simulink model "energy_aware_controller_v2"  (R2020b)
settings: Solver=VariableStepAuto  StartTime=0.0  StopTime=42  RelTol=1e-3
values from neighbouring files (symbols this model uses):
  b0 = 2 * sqrt(k0 * m_R)    [compliance_PLUS_energy_setup.m]    (also in compliance_adjusting_setup.m = 2; energy_aware_setup.m = 20; optim_criteria.m = 0.2; plot_meshes.m = 0.2)
  E_max = 1    [compliance_PLUS_energy_setup.m]    (also in energy_aware_setup.m = 0.7; optim_criteria.m = 0.5; plot_meshes.m = 0.5; setup.m)
  k0 = 20    [compliance_PLUS_energy_setup.m]    (also in compliance_adjusting_setup.m = 10; energy_aware_setup.m = 100; optim_criteria.m = 1; plot_meshes.m = 1)
  km = 100    [compliance_PLUS_energy_setup.m]    (also in compliance_adjusting_setup.m; energy_aware_setup.m; setup.m)
  m_R = 1    [compliance_PLUS_energy_setup.m]    (also in compliance_adjusting_setup.m; energy_aware_setup.m; setup.m)
  P_max = 1    [compliance_PLUS_energy_setup.m]    (also in energy_aware_setup.m = 0.2; optim_criteria.m = 0.5; plot_meshes.m = 0.5; setup.m = 0.1)
  s0 = 5    [compliance_PLUS_energy_setup.m]    (also in energy_aware_setup.m; setup.m)
  t_collision = 20    [compliance_PLUS_energy_setup.m]    (also in compliance_adjusting_setup.m; energy_aware_setup.m; setup.m)
  t_init = 2    [compliance_PLUS_energy_setup.m]    (also in compliance_adjusting_setup.m; energy_aware_setup.m; setup.m)
  x_O = 0.5    [compliance_PLUS_energy_setup.m]    (also in compliance_adjusting_setup.m; energy_aware_setup.m; setup.m)
  x_O2 = -2    [compliance_PLUS_energy_setup.m]    (also in compliance_adjusting_setup.m)
  x_R = 0    [compliance_PLUS_energy_setup.m]    (also in compliance_adjusting_setup.m; energy_aware_setup.m; setup.m)
settings Model: Creator=kika  LastModifiedBy=kika

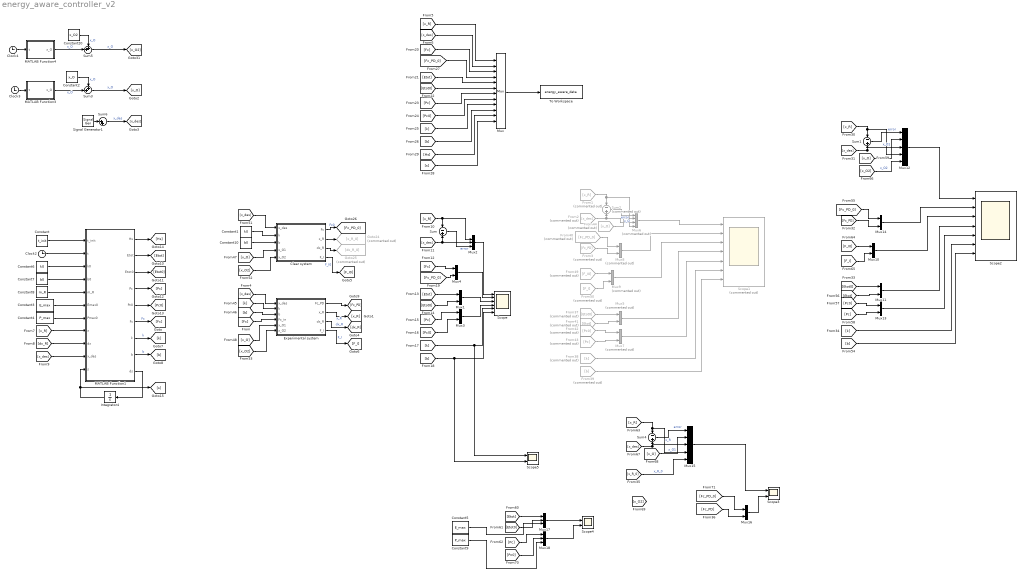
== system energy_aware_controller_v2 ==
  Clear system : Subsystem
  Clock2 : Clock
  Clock3 : Clock
  Clock4 : Clock
  Constant : Constant  Value=t_init
  Constant1 : Constant  Value=k0
  Constant10 : Constant  Value=b0
  Constant2 : Constant  Value=x_O
  Constant20 : Constant  Value=x_O2
  Constant3 : Constant  Value=E_max
  Constant4 : Constant  Value=P_max
  Constant5 : Constant  Value=E_max
  Constant6 : Constant  Value=k0
  Constant7 : Constant  Value=b0
  Constant8 : Constant  Value=m_R
  Constant9 : Constant  Value=P_max
  Experimental system : Subsystem
  From1 : From  Commented=on  GotoTag=x_R
  From2 : From  Commented=on  GotoTag=x_des
  From3 : From  Commented=on  GotoTag=Fc_PD
  From37 : From  Commented=on  GotoTag=Etot0
  From38 : From  Commented=on  GotoTag=k
  From39 : From  Commented=on  GotoTag=b
  From40 : From  Commented=on  GotoTag=Fc_PD_0
  From41 : From  Commented=on  GotoTag=Etot
  From42 : From  Commented=on  GotoTag=Pc0
  From43 : From  Commented=on  GotoTag=Pc
  From44 : From  Commented=on  GotoTag=x_O
  From49 : From  Commented=on  GotoTag=F_I0
  From50 : From  Commented=on  GotoTag=F_I
  Goto24 : Goto  Commented=on  GotoTag=x_R_0
  Goto25 : Goto  Commented=on  GotoTag=dx_R_0
  Integrator4 : Integrator  InitialCondition=s0
  MATLAB Function1 : MATLAB Function  TreatAsAtomicUnit=on
  MATLAB Function3 : MATLAB Function  TreatAsAtomicUnit=on
  MATLAB Function4 : MATLAB Function  TreatAsAtomicUnit=on
  Mux : Mux  Inputs=12
  Mux{1,3..4,10..11,13..14,16} (8 alike) : Mux  Inputs=2
  Mux12 : Mux  Inputs=5
  Mux15 : Mux  Inputs=5
  Mux17 : Mux  Inputs=3
  Mux18 : Mux  Inputs=3
  Mux2 : Mux  Inputs=3
  Mux{5,7..9} (4 alike) : Mux  Commented=on  Inputs=2
  Mux6 : Mux  Commented=on
  Scope : Scope  NumInputPorts=6
  Scope1 : Scope  Commented=on  NumInputPorts=7
  Scope2 : Scope  NumInputPorts=7
  Scope3 : Scope  NumInputPorts=2
  Scope4 : Scope  NumInputPorts=2
  Scope5 : Scope  NumInputPorts=2
  Signal Generator1 : SignalGenerator  Frequency=0.5  Units=rad/sec
  Sum : Sum  Inputs=-+
  Sum1 : Sum  Inputs=-+
  Sum2 : Sum  Commented=on  Inputs=-+
  Sum3 : Sum  Inputs=++|
  Sum4 : Sum  Inputs=-+
  Sum5 : Sum  Inputs=++|
  Sum6 : Sum  Inputs=|++
  To Workspace : ToWorkspace  VariableName=energy_aware_data  SaveFormat=Timeseries  SampleTime=-1
  wires:
  Constant4/1 -> MATLAB Function1/7(Pmax0)
  Constant3/1 -> MATLAB Function1/6(Emax0)
  MATLAB Function1/9(ds) -> Integrator4/1
  Constant7/1 -> MATLAB Function1/4(b0)
  MATLAB Function1/7(k) -> [k]  "k"
  Constant8/1 -> MATLAB Function1/5(m_R)
  Constant6/1 -> MATLAB Function1/3(k0)
  Integrator4/1 -> MATLAB Function1/11(s), [s]
  Clock2/1 -> MATLAB Function1/2(t)
  MATLAB Function1/8(b) -> [b]  "b"
  Constant/1 -> MATLAB Function1/1(t_init)
  MATLAB Function1/6(Fc) -> [Fc]  "Fc"
  [dx_R] -> MATLAB Function1/9(dx)
  [x_R] -> MATLAB Function1/8(x)
  [x_des] -> MATLAB Function1/10(x_des)
  [x_R] -> Sum/1, Mux2/1
  [x_des] -> Mux2/2, Sum/2
  Mux2/1 -> Scope/1
  [Fc] -> Mux4/1
  MATLAB Function1/5(Pc0) -> [Pc0]
  MATLAB Function1/4(Pc) -> [Pc]
  MATLAB Function1/3(Etot0) -> [Etot0]
  MATLAB Function1/2(Etot) -> [Etot]
  MATLAB Function1/1(Hs) -> [Hs]
  [Etot] -> Mux1/1
  [Etot0] -> Mux1/2
  [Pc0] -> Mux3/2
  [Pc] -> Mux3/1
  Mux1/1 -> Scope/3
  Mux3/1 -> Scope/4
  [k] -> Scope5/1, Scope/5
  [b] -> Scope5/2, Scope/6
  [Fc_PD_0] -> Mux4/2
  Mux4/1 -> Scope/2
  Sum/1 -> Mux2/3  "error"
  [Fc_PD_0] -> Mux/4
  [Fc] -> Mux/3
  [Etot] -> Mux/5
  [Etot0] -> Mux/6
  [x_des] -> Mux/2
  [x_R] -> Mux/1
  [Pc] -> Mux/7
  [Pc0] -> Mux/8
  [k] -> Mux/9
  [b] -> Mux/10
  Mux/1 -> To Workspace/1
  [Hs] -> Mux/11
  [s] -> Mux/12
  From37/1 -> Mux5/1
  Mux7/1 -> Scope1/5
  Mux8/1 -> Scope1/2
  Mux6/1 -> Scope1/1
  From43/1 -> Mux7/2
  Mux9/1 -> Scope1/3
  From42/1 -> Mux7/1
  From1/1 -> Mux6/4, Sum2/1
  From50/1 -> Mux9/2
  From41/1 -> Mux5/2
  From40/1 -> Mux8/1
  From49/1 -> Mux9/1
  From38/1 -> Scope1/6
  From39/1 -> Scope1/7
  Sum2/1 -> Mux6/1  "error"
  From3/1 -> Mux8/2
  Mux5/1 -> Scope1/4
  From44/1 -> Mux6/2  "x_O"
  From2/1 -> Mux6/3, Sum2/2
  Sum6/1 -> [x_des]  "x_des"
  Clock4/1 -> MATLAB Function4/1(t)
  Clock3/1 -> MATLAB Function3/1(t)
  Constant20/1 -> Sum5/1  "x_O"
  MATLAB Function4/1(x_O) -> Sum5/2  "x_O"
  MATLAB Function3/1(x_O) -> Sum3/2  "x_O"
  Sum5/1 -> [x_O2]  "x_O"
  Constant2/1 -> Sum3/1  "x_O"
  Sum3/1 -> [x_O]  "x_O"
  Signal Generator1/1 -> Sum6/1
  Constant10/1 -> Clear system/3(b)
  Constant1/1 -> Clear system/2(k)
  [b] -> Experimental system/3(b)
  [x_des] -> Clear system/1(x_des)
  Clear system/3(dx_R) -> Goto25/1
  [x_des] -> Experimental system/1(x_des)
  [k] -> Experimental system/2(k)
  Clear system/1(Fc) -> [Fc_PD_0]  "Fc0"
  Experimental system/3(dx_R) -> [dx_R]  "dx_R"
  Clear system/4(F_I) -> [F_I0]  "F_I0"
  [x_O2] -> Experimental system/6(x_O2)
  [Fc] -> Experimental system/4(Fc_in)
  [x_O] -> Experimental system/5(x_O1)
  [x_O] -> Clear system/4(x_O1)
  [x_O2] -> Clear system/5(x_O2)
  Clear system/2(x_R) -> Goto24/1
  Experimental system/1(Fc_PD) -> [Fc_PD]
  Experimental system/2(x_R) -> [x_R]  "x_R"
  Experimental system/4(F_I) -> [F_I]  "F_I"
  Mux14/1 -> Scope2/2
  [x_R] -> Mux12/4, Sum1/1
  Mux12/1 -> Scope2/1
  [b] -> Scope2/7
  [Pc] -> Mux13/2
  [F_I] -> Mux10/2
  Sum1/1 -> Mux12/1  "error"
  [F_I0] -> Mux10/1
  [x_des] -> Mux12/3, Sum1/2
  [x_O2] -> Mux12/5  "x_O2"
  [x_O] -> Mux12/2  "x_O1"
  [k] -> Scope2/6
  [Etot] -> Mux11/2
  Mux13/1 -> Scope2/5
  [Fc_PD] -> Mux14/2
  [Pc0] -> Mux13/1
  Mux11/1 -> Scope2/4
  [Fc_PD_0] -> Mux14/1
  Mux10/1 -> Scope2/3
  [Etot0] -> Mux11/1
  [x_R] -> Mux15/4, Sum4/1  "x_R"
  [x_O] -> Mux15/2  "x_O1"
  Sum4/1 -> Mux15/1  "error"
  Mux15/1 -> Scope3/1
  [x_des] -> Mux15/3, Sum4/2
  [Fc_PD_0] -> Mux16/1
  [x_R_0] -> Mux15/5  "x_R_0"
  [Fc_PD] -> Mux16/2
  Mux16/1 -> Scope3/2
  Mux18/1 -> Scope4/2
  [Pc0] -> Mux18/2
  [Etot] -> Mux17/1
  [Etot0] -> Mux17/2
  Mux17/1 -> Scope4/1
  [Pc] -> Mux18/1
  Constant5/1 -> Mux17/3
  Constant9/1 -> Mux18/3

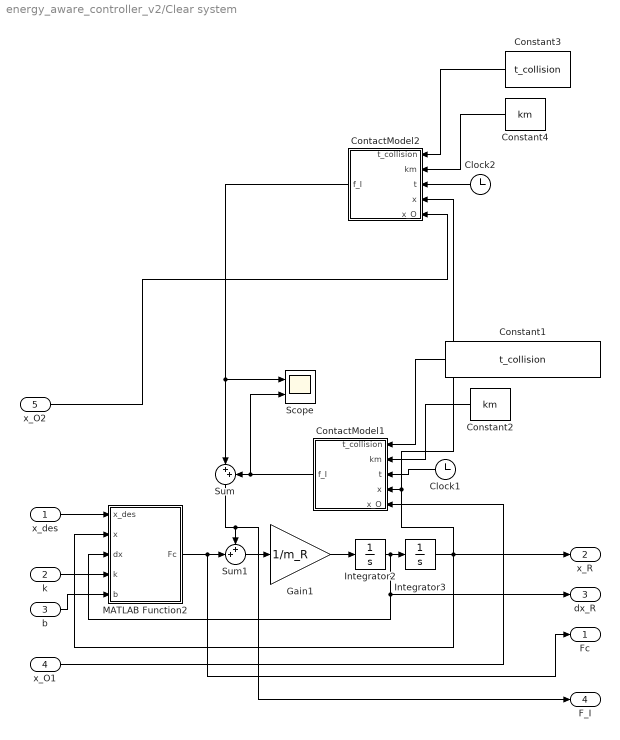
== system energy_aware_controller_v2/Clear system ==
  x_des : Inport
  k : Inport  Port=2
  b : Inport  Port=3
  x_O1 : Inport  Port=4
  x_O2 : Inport  Port=5
  Clock1 : Clock
  Clock2 : Clock
  Constant1 : Constant  Value=t_collision
  Constant2 : Constant  Value=km
  Constant3 : Constant  Value=t_collision
  Constant4 : Constant  Value=km
  ContactModel1 : MATLAB Function  TreatAsAtomicUnit=on
  ContactModel2 : MATLAB Function  TreatAsAtomicUnit=on
  Gain1 : Gain  Gain=1/m_R
  Integrator2 : Integrator
  Integrator3 : Integrator  InitialCondition=x_R
  MATLAB Function2 : MATLAB Function  TreatAsAtomicUnit=on
  Scope : Scope  NumInputPorts=2
  Sum : Sum  Inputs=|++
  Sum1 : Sum  Inputs=++|
  Fc : Outport
  x_R : Outport  Port=2
  dx_R : Outport  Port=3
  F_I : Outport  Port=4
  wires:
  k/1 -> MATLAB Function2/4(k)
  ContactModel1/1(f_I) -> Scope/2, Sum/2
  Clock1/1 -> ContactModel1/3(t)
  x_des/1 -> MATLAB Function2/1(x_des)
  b/1 -> MATLAB Function2/5(b)
  Sum1/1 -> Gain1/1
  x_O1/1 -> ContactModel1/5(x_O)
  Gain1/1 -> Integrator2/1
  MATLAB Function2/1(Fc) -> Fc/1, Sum1/2
  Integrator2/1 -> dx_R/1, MATLAB Function2/3(dx), Integrator3/1
  Constant1/1 -> ContactModel1/1(t_collision)
  Constant2/1 -> ContactModel1/2(km)
  Constant3/1 -> ContactModel2/1(t_collision)
  Integrator3/1 -> x_R/1, ContactModel2/4(x), ContactModel1/4(x), MATLAB Function2/2(x)
  x_O2/1 -> ContactModel2/5(x_O)
  Constant4/1 -> ContactModel2/2(km)
  Clock2/1 -> ContactModel2/3(t)
  Sum/1 -> F_I/1, Sum1/1
  ContactModel2/1(f_I) -> Sum/1, Scope/1

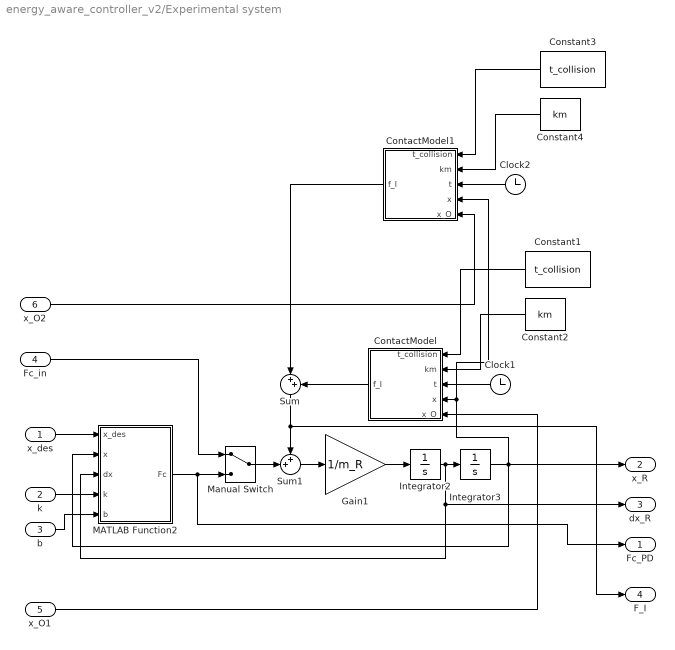
== system energy_aware_controller_v2/Experimental system ==
  x_des : Inport
  k : Inport  Port=2
  b : Inport  Port=3
  Fc_in : Inport  Port=4
  x_O1 : Inport  Port=5
  x_O2 : Inport  Port=6
  Clock1 : Clock
  Clock2 : Clock
  Constant1 : Constant  Value=t_collision
  Constant2 : Constant  Value=km
  Constant3 : Constant  Value=t_collision
  Constant4 : Constant  Value=km
  ContactModel : MATLAB Function  TreatAsAtomicUnit=on
  ContactModel1 : MATLAB Function  TreatAsAtomicUnit=on
  Gain1 : Gain  Gain=1/m_R
  Integrator2 : Integrator
  Integrator3 : Integrator  InitialCondition=x_R
  MATLAB Function2 : MATLAB Function  TreatAsAtomicUnit=on
  Manual Switch : ManualSwitch
  Sum : Sum  Inputs=|++
  Sum1 : Sum  Inputs=++|
  Fc_PD : Outport
  x_R : Outport  Port=2
  dx_R : Outport  Port=3
  F_I : Outport  Port=4
  wires:
  k/1 -> MATLAB Function2/4(k)
  ContactModel/1(f_I) -> Sum/2
  Clock1/1 -> ContactModel/3(t)
  Integrator3/1 -> x_R/1, ContactModel1/4(x), ContactModel/4(x), MATLAB Function2/2(x)
  x_des/1 -> MATLAB Function2/1(x_des)
  b/1 -> MATLAB Function2/5(b)
  Sum1/1 -> Gain1/1
  x_O1/1 -> ContactModel/5(x_O)
  Gain1/1 -> Integrator2/1
  MATLAB Function2/1(Fc) -> Manual Switch/2, Fc_PD/1
  Integrator2/1 -> dx_R/1, MATLAB Function2/3(dx), Integrator3/1
  Constant1/1 -> ContactModel/1(t_collision)
  Constant2/1 -> ContactModel/2(km)
  Fc_in/1 -> Manual Switch/1
  Manual Switch/1 -> Sum1/2
  ContactModel1/1(f_I) -> Sum/1
  Constant4/1 -> ContactModel1/2(km)
  Constant3/1 -> ContactModel1/1(t_collision)
  Clock2/1 -> ContactModel1/3(t)
  x_O2/1 -> ContactModel1/5(x_O)
  Sum/1 -> F_I/1, Sum1/1

== matlab function energy_aware_controller_v2/MATLAB Function4 ==
  data: t input; x_O output
function x_O = fcn(t)

    x_O = 0;
    if t > 56 && t < 65
        x_O = sin(0.5 * t + pi) + 0.5;
    end
    if t > 71 && t < 85
        x_O = 1.5;
    end
%     if t >= 44.5 && t < 46.8
%         x_O = 3*sin(1.5 * t - pi/4);
%     end

== matlab function energy_aware_controller_v2/Experimental system/ContactModel1 ==
  data: t_collision input; km input; t input; f_I output; x input; x_O input
function f_I = fcn(t_collision, km, t, x, x_O)


f_I = 0;

if t > t_collision
    if x < x_O
        f_I = km * (x_O - x);
    end
end

== matlab function energy_aware_controller_v2/Experimental system/MATLAB Function2 ==
  data: x_des input; Fc output; x input; dx input; k input; b input
function Fc = fcn(x_des, x, dx, k, b)

Fc = k * (x_des - x) - b * dx;

== matlab function energy_aware_controller_v2/Experimental system/ContactModel ==
  data: t_collision input; km input; t input; f_I output; x input; x_O input
function f_I = fcn(t_collision, km, t, x, x_O)


f_I = 0;

if t > t_collision
    if x > x_O
        f_I = km * (x_O - x);
    end
end

% if t > t_collision
%     if abs(x) - abs(x_O) > 0
%         f_I = km * (abs(x_O) - abs(x));
%     end
% end

== matlab function energy_aware_controller_v2/MATLAB Function3 ==
  data: t input; x_O output
function x_O = fcn(t)

    offset = -0.3;
    x_O = 1;
    if t > 23 && t < 35
        x_O = sin(0.5 * t + pi);
    end
    if t >= offset + 44.5 && t < offset +46.8
        x_O = 2*sin(1.5 * t - pi/6);
    end
    if t > 85
        x_O = 0.2;
    end

== matlab function energy_aware_controller_v2/MATLAB Function1 ==
  data: t_init input; t input; k0 input; b0 input; m_R input; Hs output; Emax0 input; Pmax0 input; Etot output; Etot0 output; Pc output; Pc0 output; Fc output; x input; k output; b output; dx input; x_des input; s input; ds output
function [Hs, Etot, Etot0, Pc, Pc0, Fc, k, b, ds] = energy_aware(t_init,t, k0, b0, m_R, Emax0, Pmax0, x, dx, x_des, s)
    
    % initialisation time
    Emax = 1000;
    Pmax = 2000;
    if t > t_init
        Emax = Emax0;
        Pmax = Pmax0;
    end

    e = x_des - x;  % control error
    
    % Kinetic energy
    T = 0.5 * m_R * dx^2;

    % stiffness abjusting using initial Potential energy
    V0 = 0.5 * k0 * e^2;
    Etot0 = T + V0;
    k = k0;
    if Etot0 > Emax
        k = (Emax - T) / (0.5 * e^2);
    end
%     if k < 0.001
%         k = 0.001;
%     end

    % damping adjusting using new stiffness
    Fs = k * e;
    Fd0 = b0 * dx;
    Fc0 = Fs - Fd0;
    Pc0 = Fc0 * dx;
    b = b0;
    if Pc0 > Pmax
        b = (Fs * dx - Pmax) / dx^2;
    end

    % new control
    Fd = b * dx;
    Fc = Fs - Fd; % control without passivity

    % adjusted total Energy and Power
    V = 0.5 * k * e^2;
    Etot = T + V;
    Pc = Fc * dx;

    % Passivity
    eps = 0.1;
    Hs = 0.5 * s^2;

    u = -Fc * s / sqrt(2 * eps);    % or u = 0;
    if Hs >= eps || Pc < 0
        u = - Fc / s;
    end

    % total contol with passivity
    Fc = -u * s;
    ds = u * dx;

== matlab function energy_aware_controller_v2/Clear system/MATLAB Function2 ==
  data: x_des input; Fc output; x input; dx input; k input; b input
function Fc = fcn(x_des, x, dx, k, b)

Fc = k * (x_des - x) - b * dx;

== matlab function energy_aware_controller_v2/Clear system/ContactModel1 ==
  data: t_collision input; km input; t input; f_I output; x input; x_O input
function f_I = fcn(t_collision, km, t, x, x_O)


f_I = 0;

if t > t_collision
    if x > x_O
        f_I = km * (x_O - x);    
    end
end

% if t > t_collision
%     if abs(x) - abs(x_O) > 0
%         f_I = km * (abs(x_O) - abs(x));
%     end
% end

== matlab function energy_aware_controller_v2/Clear system/ContactModel2 ==
  data: t_collision input; km input; t input; f_I output; x input; x_O input
function f_I = fcn(t_collision, km, t, x, x_O)


f_I = 0;


if t > t_collision
    if x < x_O
        f_I = km * (x_O - x);
    end
end
